simulink model "AbsTimeStamp"  (R2012b)
settings: Solver=FixedStepDiscrete  StartTime=0.0  StopTime=50  RelTol=1e-3
InitFcn:
  | N=256;
  | Fs = 1000;
  | bw = 5.6;
settings Model: RequirementInfo={'other' '..\..\requirements\ebd_srs.doc' '@Simulink_requirement_item_22' 'true' 'Simulink_requirement_item_22' 'Requirement' } %GIDa_f9b6cecd_8555_4b34_8c0d_e0986fea8b35  Creator=aanantha  LastModifiedBy=klindqvi
settings DataIOCC: SaveFormat=Structure  SignalLoggingSaveFormat=ModelDataLogs  SaveOutput=off  SaveTime=off  SignalLoggingName=logsOut
settings OptimizationCC: InlineParams=on  OptimizeModelRefInitCode=on  LifeSpan=1
settings DebuggingCC: ReadBeforeWriteMsg=DisableAll  WriteAfterWriteMsg=DisableAll  WriteAfterReadMsg=DisableAll  SolverPrmCheckMsg=none  InheritedTsInSrcMsg=none  ParameterPrecisionLossMsg=none  FcnCallInpInsideContextMsg=EnableAllAsWarning
settings HardwareCC: ProdLargestAtomicInteger=Long  ProdLargestAtomicFloat=Double  ProdEndianess=LittleEndian  ProdHWDeviceType=ARM Compatible->ARM Cortex
settings RTWCC: SystemTargetFile=ert.tlc  TemplateMakefile=ert_default_tmf  Description=Embedded Coder  GenerateReport=on  RTWVerbose=off  ProcessScript=ert_make_rtw_hook  IncludeHyperlinkInReport=on  LaunchReport=on  PortableWordSizes=on  CodeProfilingSaveOptions=AllData  GenerateTraceInfo=on  GenerateTraceReportSl=on  GenerateTraceReportSf=on  GenerateTraceReportEml=on  GenerateCodeMetricsReport=on
settings CodeAppCC: IgnoreCustomStorageClasses=off
settings ERTTargetCC: CodeReplacementLibrary=GCC ARM Cortex-A8  MultiwordLength=2048  GenerateSampleERTMain=on  ERTCustomFileTemplate=example_file_process.tlc  ConvertIfToSwitch=off  SuppressUnreachableDefaultCases=off

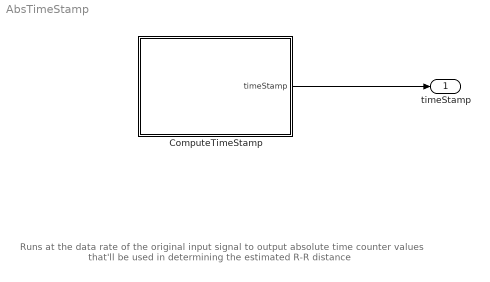
== system AbsTimeStamp ==
  note: Runs at the data rate of the original input signal
      | to output absolute time counter values that'll be used in
      | determining the estimated R-R distance
  ComputeTimeStamp : Subsystem
  timeStamp : Outport  OutDataTypeStr=uint32  PortDimensions=1  SampleTime=[0.001,0]
  wires:
  ComputeTimeStamp/1(timeStamp) -> timeStamp/1

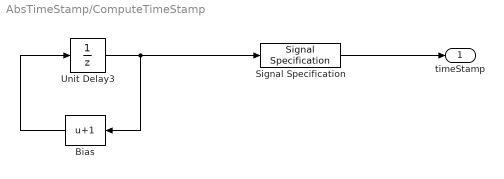
== system AbsTimeStamp/ComputeTimeStamp ==
  Bias : Bias  Bias=1
  Signal Specification : SignalSpecification  OutDataTypeStr=uint32
  Unit Delay3 : UnitDelay  SampleTime=1/Fs
  timeStamp : Outport
  wires:
  Unit Delay3/1 -> Bias/1, Signal Specification/1
  Bias/1 -> Unit Delay3/1
  Signal Specification/1 -> timeStamp/1
